simulink model "Simulation_2018b_old"  (R2018b)
settings: Solver=FixedStepAuto  StartTime=0.0  StopTime=double(Tsim)  FixedStep=param.tSample  RelTol=1e-3
StopFcn:
  | run animation
  | run plotSol
values from neighbouring files (symbols this model uses):
  grampc = grampc_update_struct_grampc(grampc,user)    [initData.m]
  param = load_parameter(param,grampc)    [script_Simulation.m]
undefined symbols (not defined in the file or in its folder): cost
settings Model: Creator=msdirauf  LastModifiedBy=Khaled
settings DataIOCC: LimitDataPoints=on  SaveFormat=Array
settings OptimizationCC: ExpressionDepthLimit=2147483647  LifeSpan=inf
settings DebuggingCC: UnderspecifiedInitializationDetection=Classic  MergeDetectMultiDrivingBlocksExec=none  SolverPrmCheckMsg=warning  StateNameClashWarn=warning  SFUnexpectedBacktrackingDiag=warning  SFNoUnconditionalDefaultTransitionDiag=warning  SFExecutionAtInitializationDiag=none
settings HardwareCC: ProdBitPerPointer=32  ProdBitPerSizeT=32  ProdBitPerPtrDiffT=32  ProdLargestAtomicFloat=None  ProdIntDivRoundTo=Undefined  ProdEndianess=Unspecified  ProdWordSize=32  ProdHWDeviceType=32-bit Generic
settings ModelReferenceCC: PropagateSignalLabelsOutOfModel=off
settings SFSimCC: SimUseLocalCustomCode=off
settings RTWCC: RTWUseLocalCustomCode=off
settings CodeAppCC: StateflowObjectComments=on
settings GRTTargetCC: TargetLangStandard=C89/C90 (ANSI)
settings ConfigComp: CovMetricSettings=dw  CovSaveCumulativeToWorkspaceVar=on  CovSaveSingleToWorkspaceVar=on  CovExternalEMLEnable=off

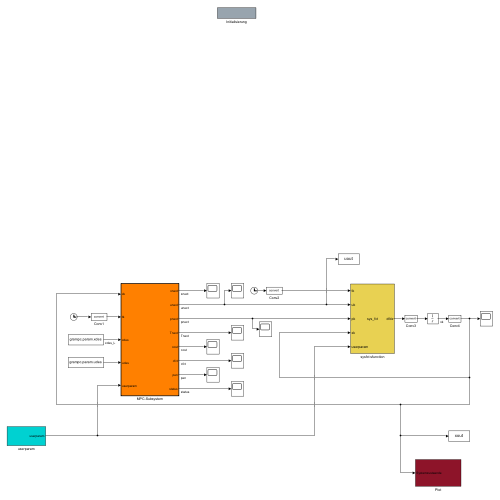
[thumbnail: Simulink's stored preview of the top-level diagram]
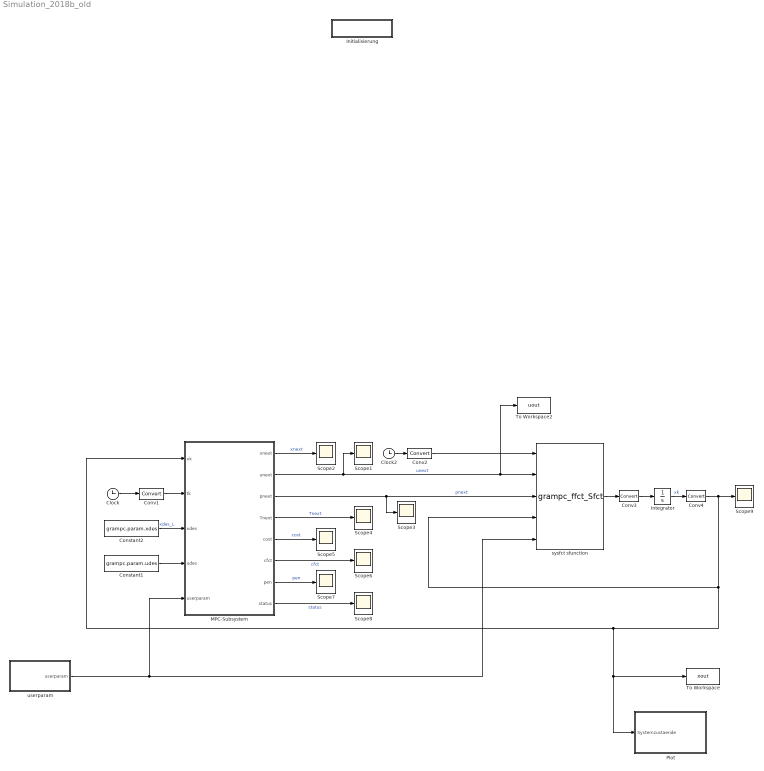
== system Simulation_2018b_old ==
  Clock : Clock
  Clock2 : Clock
  Constant1 : Constant  Value=grampc.param.udes
  Constant2 : Constant  Value=grampc.param.xdes
  Conv{1..4} (4 alike) : DataTypeConversion
  Initialisierung : Subsystem
      settings: OpenFcn=run script_Simulation
  Integrator : Integrator  InitialCondition=double(grampc.param.x0)
  MPC-Subsystem : Subsystem  TreatAsAtomicUnit=on  SystemSampleTime=double(grampc.param.dt)
  Plot : Subsystem
  Scope{1..9} (9 alike) : Scope
  To Workspace : ToWorkspace  VariableName=xout  SaveFormat=Timeseries  SampleTime=-1
  To Workspace2 : ToWorkspace  VariableName=uout  SaveFormat=Timeseries  SampleTime=-1
  sysfct sfunction : S-Function  FunctionName=grampc_ffct_Sfct  SFunctionDeploymentMode=off  EnableBusSupport=off
      mask Display:
      | port_label('input',1,'tk')
      | port_label('input',2,'uk')
      | port_label('input',3,'pk')
      | port_label('input',4,'xk')
      | port_label('input',5,'userparam')
      | 
      | port_label('output',1,'dfdx')
      | 
      | 
      | disp('sys_fct')
  userparam : Subsystem
  wires:
  Constant1/1 -> MPC-Subsystem/4(udes)
  Conv4/1 -> Plot/1(Systemzustaende), To Workspace/1, MPC-Subsystem/1(xk), sysfct sfunction/4, Scope9/1
  MPC-Subsystem/3(pnext) -> sysfct sfunction/3, Scope3/1  "pnext"
  Conv2/1 -> sysfct sfunction/1
  MPC-Subsystem/8(status) -> Scope8/1  "status"
  Integrator/1 -> Conv4/1  "xk"
  MPC-Subsystem/6(cfct) -> Scope6/1  "cfct"
  MPC-Subsystem/4(Tnext) -> Scope4/1  "Tnext"
  Conv3/1 -> Integrator/1
  MPC-Subsystem/5(cost) -> Scope5/1  "cost"
  Clock2/1 -> Conv2/1
  MPC-Subsystem/1(xnext) -> Scope2/1  "xnext"
  MPC-Subsystem/2(unext) -> Scope1/1, To Workspace2/1, sysfct sfunction/2  "unext"
  sysfct sfunction/1 -> Conv3/1
  MPC-Subsystem/7(pen) -> Scope7/1  "pen"
  Clock/1 -> Conv1/1
  userparam/1(userparam) -> sysfct sfunction/5, MPC-Subsystem/5(userparam)
  Constant2/1 -> MPC-Subsystem/3(xdes)  "xdes_L"
  Conv1/1 -> MPC-Subsystem/2(tk)

== system Simulation_2018b_old/Initialisierung ==

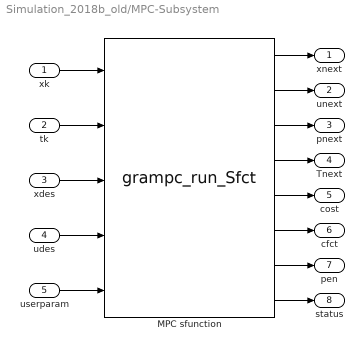
== system Simulation_2018b_old/MPC-Subsystem ==
  xk : Inport
  tk : Inport  Port=2
  xdes : Inport  Port=3
  udes : Inport  Port=4
  userparam : Inport  Port=5
  MPC sfunction : S-Function  FunctionName=grampc_run_Sfct  Parameters=grampc_sdata.intoptidx grampc_sdata.intopt grampc_sdata.numoptidx grampc_sdata.numopt grampc_sdata.numparamidx grampc_sdata.numparam  SFunctionDeploymentMode=off  EnableBusSupport=off
      mask Display:
      | port_label('input',1,'x0')
      | port_label('input',2,'t0')
      | port_label('input',3,'xdes')
      | port_label('input',4,'udes')
      | port_label('input',5,'userparam')
      | 
      | port_label('output',1,'xnext')
      | port_label('output',2,'unext')
      | port_label('output',3,'pnext')
      | port_label('output',4,'Tnext')
      | port_label('output',5,'cost')
      | port_label('output',6,'||cfct||')
      | port_label('output',7,'||pen||')
      | port_label('output',8,'status')
      | 
      | disp('GRAMPC')
  xnext : Outport  VectorParamsAs1DForOutWhenUnconnected=off
  unext : Outport  Port=2  VectorParamsAs1DForOutWhenUnconnected=off
  pnext : Outport  Port=3  VectorParamsAs1DForOutWhenUnconnected=off
  Tnext : Outport  Port=4  VectorParamsAs1DForOutWhenUnconnected=off
  cost : Outport  Port=5  VectorParamsAs1DForOutWhenUnconnected=off
  cfct : Outport  Port=6  VectorParamsAs1DForOutWhenUnconnected=off
  pen : Outport  Port=7  VectorParamsAs1DForOutWhenUnconnected=off
  status : Outport  Port=8  VectorParamsAs1DForOutWhenUnconnected=off
  wires:
  xk/1 -> MPC sfunction/1
  MPC sfunction/1 -> xnext/1
  MPC sfunction/8 -> status/1
  MPC sfunction/7 -> pen/1
  xdes/1 -> MPC sfunction/3
  MPC sfunction/6 -> cfct/1
  udes/1 -> MPC sfunction/4
  MPC sfunction/5 -> cost/1
  MPC sfunction/3 -> pnext/1
  MPC sfunction/4 -> Tnext/1
  MPC sfunction/2 -> unext/1
  tk/1 -> MPC sfunction/2
  userparam/1 -> MPC sfunction/5

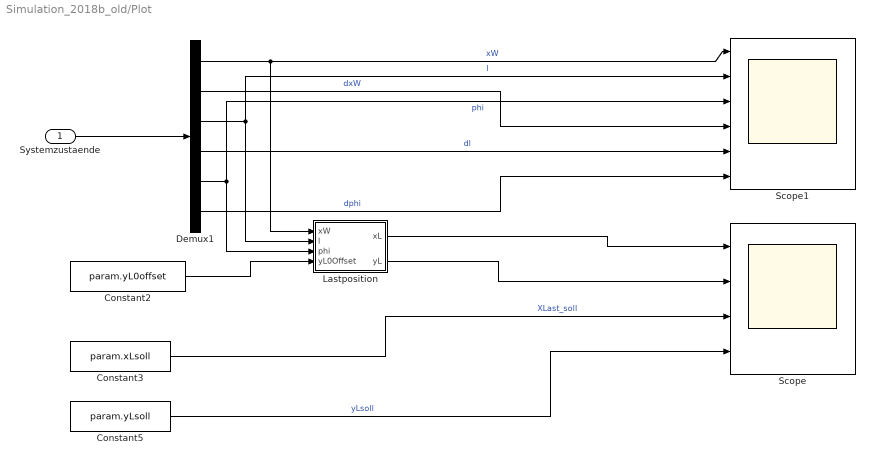
== system Simulation_2018b_old/Plot ==
  Systemzustaende : Inport
  Constant2 : Constant  Value=param.yL0offset
  Constant3 : Constant  Value=param.xLsoll
  Constant5 : Constant  Value=param.yLsoll
  Demux1 : Demux  Outputs=6
  Lastposition : MATLAB Function  TreatAsAtomicUnit=on
  Scope : Scope  NumInputPorts=4
  Scope1 : Scope  NumInputPorts=6
  wires:
  Constant5/1 -> Scope/4  "yLsoll"
  Constant3/1 -> Scope/3  "XLast_soll"
  Systemzustaende/1 -> Demux1/1
  Constant2/1 -> Lastposition/4(yL0Offset)
  Demux1/4 -> Scope1/5  "dl"
  Demux1/1 -> Lastposition/1(xW), Scope1/1  "xW"
  Demux1/3 -> Lastposition/2(l), Scope1/2  "l"
  Demux1/6 -> Scope1/6  "dphi"
  Lastposition/2(yL) -> Scope/2
  Lastposition/1(xL) -> Scope/1
  Demux1/5 -> Lastposition/3(phi), Scope1/3  "phi"
  Demux1/2 -> Scope1/4  "dxW"

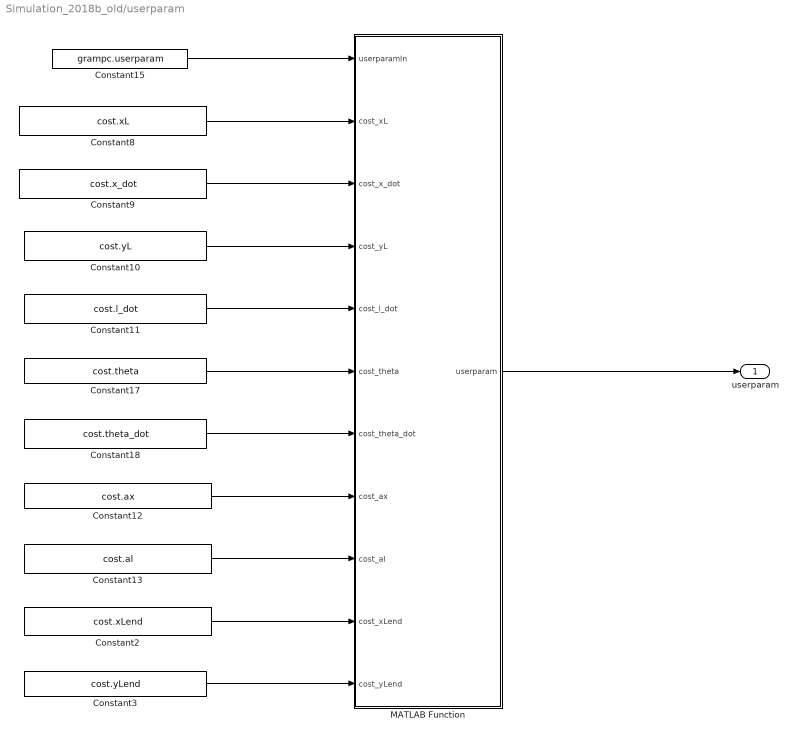
== system Simulation_2018b_old/userparam ==
  Constant10 : Constant  Value=cost.yL
  Constant11 : Constant  Value=cost.l_dot
  Constant12 : Constant  Value=cost.ax
  Constant13 : Constant  Value=cost.al
  Constant15 : Constant  Value=grampc.userparam
  Constant17 : Constant  Value=cost.theta
  Constant18 : Constant  Value=cost.theta_dot
  Constant2 : Constant  Value=cost.xLend
  Constant3 : Constant  Value=cost.yLend
  Constant8 : Constant  Value=cost.xL
  Constant9 : Constant  Value=cost.x_dot
  MATLAB Function : MATLAB Function  TreatAsAtomicUnit=on
  userparam : Outport  VectorParamsAs1DForOutWhenUnconnected=off
  wires:
  MATLAB Function/1(userparam) -> userparam/1
  Constant8/1 -> MATLAB Function/2(cost_xL)
  Constant15/1 -> MATLAB Function/1(userparamIn)
  Constant9/1 -> MATLAB Function/3(cost_x_dot)
  Constant10/1 -> MATLAB Function/4(cost_yL)
  Constant11/1 -> MATLAB Function/5(cost_l_dot)
  Constant17/1 -> MATLAB Function/6(cost_theta)
  Constant18/1 -> MATLAB Function/7(cost_theta_dot)
  Constant12/1 -> MATLAB Function/8(cost_ax)
  Constant13/1 -> MATLAB Function/9(cost_al)
  Constant2/1 -> MATLAB Function/10(cost_xLend)
  Constant3/1 -> MATLAB Function/11(cost_yLend)

== matlab function Simulation_2018b_old/Plot/Lastposition ==
  data: xW input; xL output; l input; phi input; yL output; yL0Offset input
function [xL, yL] = fcn(xW, l, phi, yL0Offset)
    
    xL = xW + sin(phi)*l;
    yL = yL0Offset - cos(phi)*l;

end

== matlab function Simulation_2018b_old/userparam/MATLAB Function ==
  data: userparamIn input; userparam output; cost_xL input; cost_x_dot input; cost_yL input; cost_l_dot input; cost_theta input; cost_theta_dot input; cost_ax input; cost_al input; cost_xLend input; cost_yLend input
function userparam   = fcn(userparamIn, cost_xL, cost_x_dot, cost_yL, cost_l_dot, ...
         cost_theta, cost_theta_dot, cost_ax, cost_al, ...
         cost_xLend, cost_yLend)

userparam = userparamIn;

userparam(1) = cost_xL;
userparam(2) = cost_x_dot;
userparam(3) = cost_yL;
userparam(4) = cost_l_dot;

userparam(5) = cost_theta;
userparam(6) = cost_theta_dot;

userparam(7) = cost_ax;
userparam(8) = cost_al;

userparam(9) = cost_xLend;
userparam(10) = cost_yLend;
